simulink subsystem "rocket_plant_combined"  (R2026a)
settings: Solver=VariableStepAuto
undefined symbols (not defined in the file): alt, angle_vert_deg, crossrange, location, sim_time, vel_vert
libraries: aerolibanim x1, simulink_extras x1
settings Model: Creator=joedo  LastModifiedBy=trist

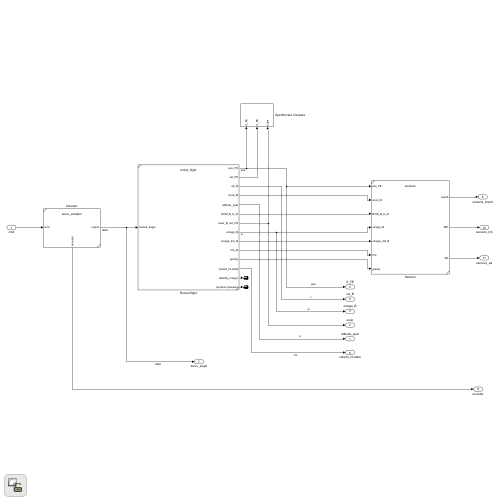
[thumbnail: Simulink's stored preview of the top-level diagram]
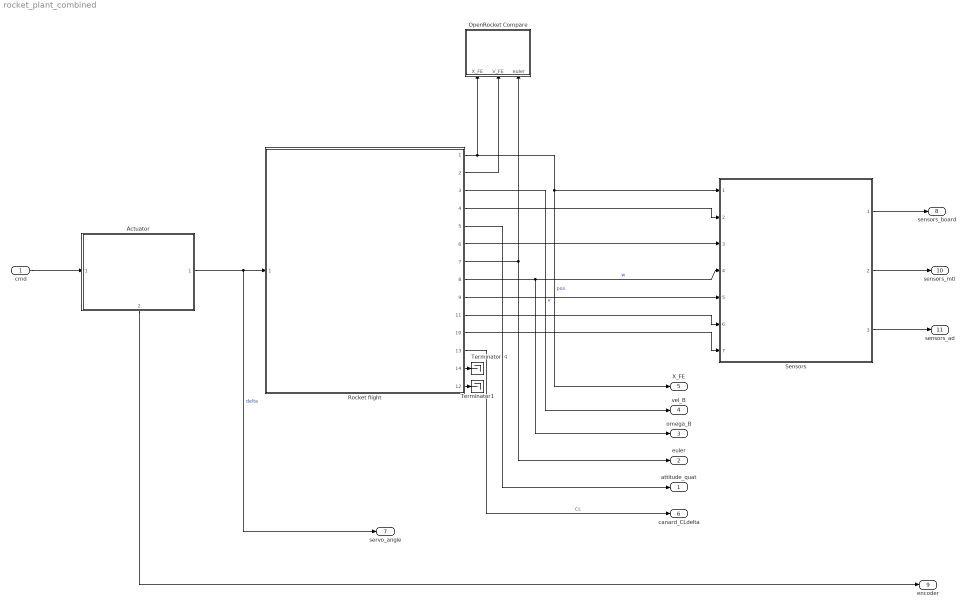
== system rocket_plant_combined ==
  cmd : Inport
  Actuator : Subsystem  ReferencedSubsystem=servo_actuator
      settings: PortSchema="{\"entries\":[{\"content\":{\"sides\":[{\"content\":{\"connectorIds\":[\"In1\"]},\"type\":\"ConnectorPlacement.EquallySpacedRectSide\",\"uuid\":\"f1fe2692-4f3a-49f6-a037-219451f9c8a9\"},{\"content\":{\"connectorIds\":[\"Out1\"],\"side\":\"RIGHT\"},\"type\":\"ConnectorPlacement.EquallySpacedRectSide\",\"uuid\":\"c09abda5-ce02-4dc4-8bf7-df22ff98c510\"},{\"content\":{\"side\":\"TOP\"},\"type\":\"ConnectorPlacement.EquallySpacedRectSide\",\"uuid\":\"d89775cf-018a-424b-8fdc-70f841ad885b\"},{\"content\":{\"connectorIds\":[\"Out2\"],\"side\":\"BOTTOM\"},\"type\":\"ConnectorPlacement.EquallySpacedRectSide\",\"uuid\":\"dc16bf3c-a1ac-4f88-a587-41692023e4d4\"}]},\"type\":\"ConnectorPlacement.EquallySpacedConnector\",\"uuid\":\"f43e876a-9b83-427e-9fa5-752c9eee6ca7\"}],\"packageUris\":[\"http://schema.mathworks.com/mf0/Connector/R2020b\"],\"version\":\"1.0\"}"
  OpenRocket Compare : Subsystem
  Rocket flight : Subsystem  ReferencedSubsystem=rocket_flight
      settings: PortSchema="{\"entries\":[{\"content\":{\"sides\":[{\"content\":{\"connectorIds\":[\"In1\"]},\"type\":\"ConnectorPlacement.EquallySpacedRectSide\",\"uuid\":\"9f79cae0-15ae-41cc-86ca-52b2ba536b20\"},{\"content\":{\"connectorIds\":[\"Out1\",\"Out2\",\"Out3\",\"Out4\",\"Out5\",\"Out6\",\"Out7\",\"Out8\",\"Out9\",\"Out11\",\"Out10\",\"Out13\",\"Out14\",\"Out12\"],\"side\":\"RIGHT\"},\"type\":\"ConnectorPlacement.EquallySpacedRectSide\",\"uuid\":\"ebcb1700-a632-4dda-8ea5-5b87e6fa3b6a\"},{\"content\":{\"side\":\"TOP\"},\"type\":\"ConnectorPlacement.EquallySpacedRectSide\",\"uuid\":\"efdf61b2-36e8-47a1-89a6-5eee4bf93d92\"}]},\"type\":\"ConnectorPlacement.EquallySpacedConnector\",\"uuid\":\"49b511cd-3c57-4668-a103-5fb675f3d38c\"}],\"packageUris\":[\"http://schema.mathworks.com/mf0/Connector/R2020b\"],\"version\":\"1.0\"}"
  Sensors : Subsystem  ReferencedSubsystem=sensors
  Terminator : Terminator
  Terminator1 : Terminator
  attitude_quat : Outport
  euler : Outport  Port=2
  omega_B : Outport  Port=3
  vel_B : Outport  Port=4
  X_FE : Outport  Port=5
  canard_CLdelta : Outport  Port=6
  servo_angle : Outport  Port=7
  sensors_board : Outport  Port=8
  encoder : Outport  Port=9  PortDimensions=1
  sensors_mti : Outport  Port=10
  sensors_ad : Outport  Port=11
  wires:
  Rocket flight/7 -> euler/1, OpenRocket Compare/3(euler)
  Rocket flight/5 -> attitude_quat/1  "q"
  Rocket flight/13 -> canard_CLdelta/1  "CL"
  Actuator/2 -> encoder/1
  Actuator/1 -> Rocket flight/1, servo_angle/1  "delta"
  cmd/1 -> Actuator/1
  Sensors/1 -> sensors_board/1
  Sensors/3 -> sensors_ad/1
  Sensors/2 -> sensors_mti/1
  Rocket flight/1 -> OpenRocket Compare/1(X_FE), Sensors/1, X_FE/1  "pos"
  Rocket flight/8 -> Sensors/4, omega_B/1  "w"
  Rocket flight/6 -> Sensors/3
  Rocket flight/9 -> Sensors/5
  Rocket flight/10 -> Sensors/7
  Rocket flight/11 -> Sensors/6
  Rocket flight/4 -> Sensors/2
  Rocket flight/3 -> vel_B/1  "v"
  Rocket flight/2 -> OpenRocket Compare/2(V_FE)
  Rocket flight/14 -> Terminator/1
  Rocket flight/12 -> Terminator1/1

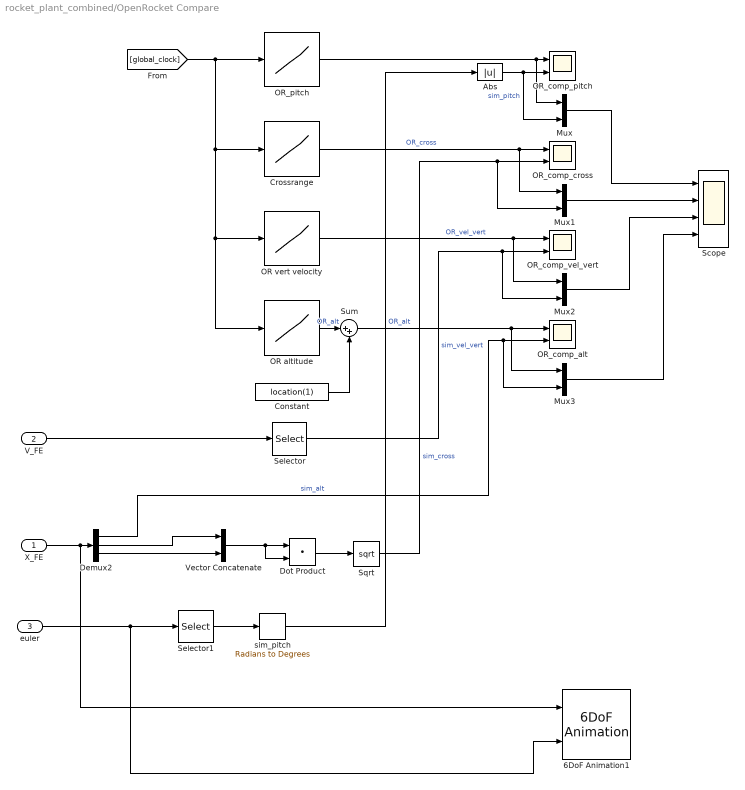
== system rocket_plant_combined/OpenRocket Compare ==
  X_FE : Inport
  V_FE : Inport  Port=2
  euler : Inport  Port=3
  6DoF Animation1 : aerolibanim/6DoF Animation  u1=[0 8000 -100 100 0 400]  u2=0.1  u3=5  u4=[location(1)-5 0 0]  u5=Fly alongside  u6=[-50 20 0]  u7=10  u8=off
  Abs : Abs  SaturateOnIntegerOverflow=off
  Constant : Constant  Value=location(1)
  Crossrange : Lookup_n-D  NumberOfTableDimensions=1  BreakpointsForDimension1=sim_time  Table=crossrange  InternalRulePriority=Speed  RndMeth=Simplest
  Demux2 : Demux  Outputs=3
  Dot Product : DotProduct  OutDataTypeStr=Inherit: Inherit via internal rule
  Mux{,1..3} (4 alike) : Mux  Inputs=2
  OR altitude : Lookup_n-D  NumberOfTableDimensions=1  BreakpointsForDimension1=sim_time  Table=alt  InternalRulePriority=Speed  RndMeth=Simplest
  OR vert velocity : Lookup_n-D  NumberOfTableDimensions=1  BreakpointsForDimension1=sim_time  Table=vel_vert  InternalRulePriority=Speed  RndMeth=Simplest
  OR_comp_alt : Scope  NumInputPorts=2
      settings: ActiveDisplayYMinimum=-838.88766  ActiveDisplayYMaximum=7549.94141  DataLoggingVariableName=ScopeData8
  OR_comp_cross : Scope  NumInputPorts=2
      settings: ActiveDisplayYMinimum=-199.36184  ActiveDisplayYMaximum=1794.25654  DataLoggingVariableName=ScopeData20
  OR_comp_pitch : Scope  NumInputPorts=2
      settings: ActiveDisplayYMinimum=-13.012  ActiveDisplayYMaximum=167.10802  DataLoggingVariableName=ScopeData21
  OR_comp_vel_vert : Scope  NumInputPorts=2
      settings: ActiveDisplayYMinimum=-95.80315  ActiveDisplayYMaximum=488.12758  DataLoggingVariableName=ScopeData23
  OR_pitch : Lookup_n-D  NumberOfTableDimensions=1  BreakpointsForDimension1=sim_time  Table=angle_vert_deg  InternalRulePriority=Speed  RndMeth=Simplest
  Scope : Scope  NumInputPorts=4
      settings: ActiveDisplayYMinimum=-12.605499999999971  ActiveDisplayYMaximum=113.4495  DataLoggingVariableName=ScopeData24
  Selector : Selector  InputPortWidth=3  IndexOptions=Index vector (dialog)  Indices=[1]  OutputSizes=1
  Selector1 : Selector  InputPortWidth=3  IndexOptions=Index vector (dialog)  Indices=[2]  OutputSizes=1
  Sqrt : Sqrt
  Sum : Sum  Inputs=|++
  Vector Concatenate : Concatenate
  sim_pitch : simulink_extras/Transformations/Radians to Degrees
  wires:
  sim_pitch/1 -> Abs/1
  OR vert velocity/1 -> OR_comp_vel_vert/1, Mux2/1  "OR_vel_vert"
  Crossrange/1 -> Mux1/1, OR_comp_cross/1  "OR_cross"
  Dot Product/1 -> Sqrt/1
  Demux2/1 -> OR_comp_alt/2, Mux3/2  "sim_alt"
  V_FE/1 -> Selector/1
  Selector/1 -> OR_comp_vel_vert/2, Mux2/2  "sim_vel_vert"
  Sum/1 -> Mux3/1, OR_comp_alt/1  "OR_alt"
  Mux3/1 -> Scope/4
  Mux2/1 -> Scope/3
  OR altitude/1 -> Sum/1  "OR_alt"
  Vector Concatenate/1 -> Dot Product/1, Dot Product/2
  Mux1/1 -> Scope/2
  euler/1 -> Selector1/1, 6DoF Animation1/2
  Abs/1 -> Mux/2, OR_comp_pitch/2  "sim_pitch"
  Selector1/1 -> sim_pitch/1
  X_FE/1 -> Demux2/1, 6DoF Animation1/1
  Demux2/2 -> Vector Concatenate/1
  Sqrt/1 -> OR_comp_cross/2, Mux1/2  "sim_cross"
  Mux/1 -> Scope/1
  Constant/1 -> Sum/2
  Demux2/3 -> Vector Concatenate/2
  OR_pitch/1 -> Mux/1, OR_comp_pitch/1
  [global_clock] -> OR_pitch/1, OR altitude/1, OR vert velocity/1, Crossrange/1
